simulink model "MIL4L3_SW6_V1_20220211"  (R2018b)
settings: Solver=FixedStepAuto  StartTime=0.0  StopTime=inf  FixedStep=0.001  RelTol=1e-3
PreLoadFcn:
  | A0_MILtest;
undefined symbols (not defined in the file or in its folder): Clb_ICADirect_LaneDisp_StateFive, Clb_ICADirect_LaneDisp_StateFour, Clb_ICADirect_LaneDisp_StateOne, Clb_ICADirect_LaneDisp_StateThree, Clb_ICADirect_LaneDisp_StateTwo, Clb_ICADirect_LaneDisp_StateZero, Clb_ICADirect_LaneDispSW, Clb_ICADirect_TrnLghtsCom_Switch, Clb_ICADirect_TrnLghtsCom_Value, Clb_ICADirect_TrnLghtsCrtl_Inhb, IMAP_Clb_ACU_Driver_Belt, IMAP_Clb_ACU_Driver_Belt_Over, IMAP_Clb_ACU_Passenger_Belt, IMAP_Clb_ACU_Passenger_Belt_Over, IMAP_Clb_ACU_RearLeft_Belt, IMAP_Clb_ACU_RearLeft_Belt_Over, IMAP_Clb_ACU_RearMiddle_Belt, IMAP_Clb_ACU_RearMiddle_Belt_Over, IMAP_Clb_ACU_RearRight_Belt, IMAP_Clb_ACU_RearRight_Belt_Over, IMAP_Clb_AEB_Switch, IMAP_Clb_AEB_Switch_Over, IMAP_Clb_ALC_TLC_Mode, IMAP_Clb_ALC_TLC_Mode_Over, IMAP_Clb_BCM_Battery_Voltage, IMAP_Clb_BCM_Battery_Voltage_Over, IMAP_Clb_BCM_BrakeLamp_State, IMAP_Clb_BCM_BrakeLamp_State_Over, IMAP_Clb_BCM_CHMSL_Status, IMAP_Clb_BCM_CHMSL_Status_Over, IMAP_Clb_BCM_Door_Lock_State, IMAP_Clb_BCM_Door_Lock_State_Over, IMAP_Clb_BCM_FrontWiper_State, IMAP_Clb_BCM_FrontWiper_State_Over, IMAP_Clb_BCM_FrontWiper_Switch, IMAP_Clb_BCM_FrontWiper_Switch_Over, IMAP_Clb_BCM_HazardLamp, IMAP_Clb_BCM_HazardLamp_Over, IMAP_Clb_BCM_HazardLamp_Switch, IMAP_Clb_BCM_HazardLamp_Switch_Over, IMAP_Clb_BCM_HighBeam_State, IMAP_Clb_BCM_HighBeam_State_Over, IMAP_Clb_BCM_Ignition_State, IMAP_Clb_BCM_Ignition_State_Over, IMAP_Clb_BCM_IHBC_Enabled, IMAP_Clb_BCM_IHBC_Enabled_Over, IMAP_Clb_BCM_Left_Light, IMAP_Clb_BCM_Left_Light_Over, IMAP_Clb_BCM_LeftTurn_Switch, IMAP_Clb_BCM_LeftTurn_Switch_Over, IMAP_Clb_BCM_LF_Door_State, IMAP_Clb_BCM_LF_Door_State_Over, IMAP_Clb_BCM_LowBeam_State, IMAP_Clb_BCM_LowBeam_State_Over, IMAP_Clb_BCM_LR_Door_State, IMAP_Clb_BCM_LR_Door_State_Over, IMAP_Clb_BCM_RF_Door_State, IMAP_Clb_BCM_RF_Door_State_Over, IMAP_Clb_BCM_Right_Light, IMAP_Clb_BCM_Right_Light_Over ... (+547)
libraries: CarMaker4SL x2153, simulink x292, dspstat3 x3, canmsglib x2, simulink_extras x1
(part 3 of 52)

== system MIL4L3_SW6_V1_20220211/CarMaker/VehicleControl/Radar_Define ==
  Define CM Dict : CarMaker4SL/Define CM Dict  xname=User.IO.Out.T00.dtct  xmono=off  xtype=Double4  xdvaplace=None  xnstates=0  xfirststate=0  xinitial=0
  Define CM Dict1 : CarMaker4SL/Define CM Dict  xname=User.IO.Out.T01.dtct  xmono=off  xtype=Double4  xdvaplace=None  xnstates=0  xfirststate=0  xinitial=0
  Define CM Dict10 : CarMaker4SL/Define CM Dict  xname=User.IO.Out.T02.LatDistance  xmono=off  xtype=Double4  xdvaplace=None  xnstates=0  xfirststate=0  xinitial=0
  Define CM Dict11 : CarMaker4SL/Define CM Dict  xname=User.IO.Out.T03.LatDistance  xmono=off  xtype=Double4  xdvaplace=None  xnstates=0  xfirststate=0  xinitial=0
  Define CM Dict12 : CarMaker4SL/Define CM Dict  xname=User.IO.Out.T00.RelativeLongVelo  xmono=off  xtype=Double4  xdvaplace=None  xnstates=0  xfirststate=0  xinitial=0
  Define CM Dict13 : CarMaker4SL/Define CM Dict  xname=User.IO.Out.T01.RelativeLongVelo  xmono=off  xtype=Double4  xdvaplace=None  xnstates=0  xfirststate=0  xinitial=0
  Define CM Dict14 : CarMaker4SL/Define CM Dict  xname=User.IO.Out.T02.RelativeLongVelo  xmono=off  xtype=Double4  xdvaplace=None  xnstates=0  xfirststate=0  xinitial=0
  Define CM Dict15 : CarMaker4SL/Define CM Dict  xname=User.IO.Out.T03.RelativeLongVelo  xmono=off  xtype=Double4  xdvaplace=None  xnstates=0  xfirststate=0  xinitial=0
  Define CM Dict16 : CarMaker4SL/Define CM Dict  xname=User.IO.Out.T00.RelativeLatVelo  xmono=off  xtype=Double4  xdvaplace=None  xnstates=0  xfirststate=0  xinitial=0
  Define CM Dict17 : CarMaker4SL/Define CM Dict  xname=User.IO.Out.T01.RelativeLatVelo  xmono=off  xtype=Double4  xdvaplace=None  xnstates=0  xfirststate=0  xinitial=0
  Define CM Dict18 : CarMaker4SL/Define CM Dict  xname=User.IO.Out.T02.RelativeLatVelo  xmono=off  xtype=Double4  xdvaplace=None  xnstates=0  xfirststate=0  xinitial=0
  Define CM Dict19 : CarMaker4SL/Define CM Dict  xname=User.IO.Out.T03.RelativeLatVelo  xmono=off  xtype=Double4  xdvaplace=None  xnstates=0  xfirststate=0  xinitial=0
  Define CM Dict2 : CarMaker4SL/Define CM Dict  xname=User.IO.Out.T02.dtct  xmono=off  xtype=Double4  xdvaplace=None  xnstates=0  xfirststate=0  xinitial=0
  Define CM Dict20 : CarMaker4SL/Define CM Dict  xname=User.IO.Out.T00.RelativeLatAcc  xmono=off  xtype=Double4  xdvaplace=None  xnstates=0  xfirststate=0  xinitial=0
  Define CM Dict21 : CarMaker4SL/Define CM Dict  xname=User.IO.Out.T01.RelativeLatAcc  xmono=off  xtype=Double4  xdvaplace=None  xnstates=0  xfirststate=0  xinitial=0
  Define CM Dict22 : CarMaker4SL/Define CM Dict  xname=User.IO.Out.T02.RelativeLatAcc  xmono=off  xtype=Double4  xdvaplace=None  xnstates=0  xfirststate=0  xinitial=0
  Define CM Dict23 : CarMaker4SL/Define CM Dict  xname=User.IO.Out.T03.RelativeLatAcc  xmono=off  xtype=Double4  xdvaplace=None  xnstates=0  xfirststate=0  xinitial=0
  Define CM Dict24 : CarMaker4SL/Define CM Dict  xname=User.IO.Out.T00.RelativeLongAcc  xmono=off  xtype=Double4  xdvaplace=None  xnstates=0  xfirststate=0  xinitial=0
  Define CM Dict25 : CarMaker4SL/Define CM Dict  xname=User.IO.Out.T01.RelativeLongAcc  xmono=off  xtype=Double4  xdvaplace=None  xnstates=0  xfirststate=0  xinitial=0
  Define CM Dict26 : CarMaker4SL/Define CM Dict  xname=User.IO.Out.T02.RelativeLongAcc  xmono=off  xtype=Double4  xdvaplace=None  xnstates=0  xfirststate=0  xinitial=0
  Define CM Dict27 : CarMaker4SL/Define CM Dict  xname=User.IO.Out.T03.RelativeLongAcc  xmono=off  xtype=Double4  xdvaplace=None  xnstates=0  xfirststate=0  xinitial=0
  Define CM Dict28 : CarMaker4SL/Define CM Dict  xname=User.IO.Out.T00.AbsoluteLongVelo  xmono=off  xtype=Double4  xdvaplace=None  xnstates=0  xfirststate=0  xinitial=0
  Define CM Dict29 : CarMaker4SL/Define CM Dict  xname=User.IO.Out.T01.AbsoluteLongVelo  xmono=off  xtype=Double4  xdvaplace=None  xnstates=0  xfirststate=0  xinitial=0
  Define CM Dict3 : CarMaker4SL/Define CM Dict  xname=User.IO.Out.T03.dtct  xmono=off  xtype=Double4  xdvaplace=None  xnstates=0  xfirststate=0  xinitial=0
  Define CM Dict30 : CarMaker4SL/Define CM Dict  xname=User.IO.Out.T02.AbsoluteLongVelo  xmono=off  xtype=Double4  xdvaplace=None  xnstates=0  xfirststate=0  xinitial=0
  Define CM Dict31 : CarMaker4SL/Define CM Dict  xname=User.IO.Out.T03.AbsoluteLongVelo  xmono=off  xtype=Double4  xdvaplace=None  xnstates=0  xfirststate=0  xinitial=0
  Define CM Dict32 : CarMaker4SL/Define CM Dict  xname=User.IO.Out.T00.AbsoluteLongAcc  xmono=off  xtype=Double4  xdvaplace=None  xnstates=0  xfirststate=0  xinitial=0
  Define CM Dict33 : CarMaker4SL/Define CM Dict  xname=User.IO.Out.T01.AbsoluteLongAcc  xmono=off  xtype=Double4  xdvaplace=None  xnstates=0  xfirststate=0  xinitial=0
  Define CM Dict34 : CarMaker4SL/Define CM Dict  xname=User.IO.Out.T02.AbsoluteLongAcc  xmono=off  xtype=Double4  xdvaplace=None  xnstates=0  xfirststate=0  xinitial=0
  Define CM Dict35 : CarMaker4SL/Define CM Dict  xname=User.IO.Out.T03.AbsoluteLongAcc  xmono=off  xtype=Double4  xdvaplace=None  xnstates=0  xfirststate=0  xinitial=0
  Define CM Dict36 : CarMaker4SL/Define CM Dict  xname=User.IO.Out.T00.AbsoluteLatVelo  xmono=off  xtype=Double4  xdvaplace=None  xnstates=0  xfirststate=0  xinitial=0
  Define CM Dict37 : CarMaker4SL/Define CM Dict  xname=User.IO.Out.T01.AbsoluteLatVelo  xmono=off  xtype=Double4  xdvaplace=None  xnstates=0  xfirststate=0  xinitial=0
  Define CM Dict38 : CarMaker4SL/Define CM Dict  xname=User.IO.Out.T02.AbsoluteLatVelo  xmono=off  xtype=Double4  xdvaplace=None  xnstates=0  xfirststate=0  xinitial=0
  Define CM Dict39 : CarMaker4SL/Define CM Dict  xname=User.IO.Out.T03.AbsoluteLatVelo  xmono=off  xtype=Double4  xdvaplace=None  xnstates=0  xfirststate=0  xinitial=0
  Define CM Dict4 : CarMaker4SL/Define CM Dict  xname=User.IO.Out.T00.LongDistance  xmono=off  xtype=Double4  xdvaplace=None  xnstates=0  xfirststate=0  xinitial=0
  Define CM Dict40 : CarMaker4SL/Define CM Dict  xname=User.IO.Out.T00.AbsoluteLatAcc  xmono=off  xtype=Double4  xdvaplace=None  xnstates=0  xfirststate=0  xinitial=0
  Define CM Dict41 : CarMaker4SL/Define CM Dict  xname=User.IO.Out.T01.AbsoluteLatAcc  xmono=off  xtype=Double4  xdvaplace=None  xnstates=0  xfirststate=0  xinitial=0
  Define CM Dict42 : CarMaker4SL/Define CM Dict  xname=User.IO.Out.T02.AbsoluteLatAcc  xmono=off  xtype=Double4  xdvaplace=None  xnstates=0  xfirststate=0  xinitial=0
  Define CM Dict43 : CarMaker4SL/Define CM Dict  xname=User.IO.Out.T03.AbsoluteLatAcc  xmono=off  xtype=Double4  xdvaplace=None  xnstates=0  xfirststate=0  xinitial=0
  Define CM Dict44 : CarMaker4SL/Define CM Dict  xname=User.IO.Out.T00.ClassType  xmono=off  xtype=Double4  xdvaplace=None  xnstates=0  xfirststate=0  xinitial=0
  Define CM Dict45 : CarMaker4SL/Define CM Dict  xname=User.IO.Out.T01.ClassType  xmono=off  xtype=Double4  xdvaplace=None  xnstates=0  xfirststate=0  xinitial=0
  Define CM Dict46 : CarMaker4SL/Define CM Dict  xname=User.IO.Out.T02.ClassType  xmono=off  xtype=Double4  xdvaplace=None  xnstates=0  xfirststate=0  xinitial=0
  Define CM Dict47 : CarMaker4SL/Define CM Dict  xname=User.IO.Out.T03.ClassType  xmono=off  xtype=Double4  xdvaplace=None  xnstates=0  xfirststate=0  xinitial=0
  Define CM Dict48 : CarMaker4SL/Define CM Dict  xname=User.IO.Out.T00.ClassProbValue  xmono=off  xtype=Double4  xdvaplace=None  xnstates=0  xfirststate=0  xinitial=0
  Define CM Dict49 : CarMaker4SL/Define CM Dict  xname=User.IO.Out.T01.ClassProbValue  xmono=off  xtype=Double4  xdvaplace=None  xnstates=0  xfirststate=0  xinitial=0
  Define CM Dict5 : CarMaker4SL/Define CM Dict  xname=User.IO.Out.T01.LongDistance  xmono=off  xtype=Double4  xdvaplace=None  xnstates=0  xfirststate=0  xinitial=0
  Define CM Dict50 : CarMaker4SL/Define CM Dict  xname=User.IO.Out.T02.ClassProbValue  xmono=off  xtype=Double4  xdvaplace=None  xnstates=0  xfirststate=0  xinitial=0
  Define CM Dict51 : CarMaker4SL/Define CM Dict  xname=User.IO.Out.T03.ClassProbValue  xmono=off  xtype=Double4  xdvaplace=None  xnstates=0  xfirststate=0  xinitial=0
  Define CM Dict52 : CarMaker4SL/Define CM Dict  xname=User.IO.Out.T00.Length  xmono=off  xtype=Double4  xdvaplace=None  xnstates=0  xfirststate=0  xinitial=0
  Define CM Dict53 : CarMaker4SL/Define CM Dict  xname=User.IO.Out.T01.Length  xmono=off  xtype=Double4  xdvaplace=None  xnstates=0  xfirststate=0  xinitial=0
  Define CM Dict54 : CarMaker4SL/Define CM Dict  xname=User.IO.Out.T02.Length  xmono=off  xtype=Double4  xdvaplace=None  xnstates=0  xfirststate=0  xinitial=0
  Define CM Dict55 : CarMaker4SL/Define CM Dict  xname=User.IO.Out.T03.Length  xmono=off  xtype=Double4  xdvaplace=None  xnstates=0  xfirststate=0  xinitial=0
  Define CM Dict56 : CarMaker4SL/Define CM Dict  xname=User.IO.Out.T00.Widh  xmono=off  xtype=Double4  xdvaplace=None  xnstates=0  xfirststate=0  xinitial=0
  Define CM Dict57 : CarMaker4SL/Define CM Dict  xname=User.IO.Out.T01.Widh  xmono=off  xtype=Double4  xdvaplace=None  xnstates=0  xfirststate=0  xinitial=0
  Define CM Dict58 : CarMaker4SL/Define CM Dict  xname=User.IO.Out.T02.Widh  xmono=off  xtype=Double4  xdvaplace=None  xnstates=0  xfirststate=0  xinitial=0
  Define CM Dict59 : CarMaker4SL/Define CM Dict  xname=User.IO.Out.T03.Widh  xmono=off  xtype=Double4  xdvaplace=None  xnstates=0  xfirststate=0  xinitial=0
  Define CM Dict6 : CarMaker4SL/Define CM Dict  xname=User.IO.Out.T02.LongDistance  xmono=off  xtype=Double4  xdvaplace=None  xnstates=0  xfirststate=0  xinitial=0
  Define CM Dict60 : CarMaker4SL/Define CM Dict  xname=User.IO.Out.T00.Height  xmono=off  xtype=Double4  xdvaplace=None  xnstates=0  xfirststate=0  xinitial=0
  Define CM Dict61 : CarMaker4SL/Define CM Dict  xname=User.IO.Out.T01.Height  xmono=off  xtype=Double4  xdvaplace=None  xnstates=0  xfirststate=0  xinitial=0
  Define CM Dict62 : CarMaker4SL/Define CM Dict  xname=User.IO.Out.T02.Height  xmono=off  xtype=Double4  xdvaplace=None  xnstates=0  xfirststate=0  xinitial=0
  Define CM Dict63 : CarMaker4SL/Define CM Dict  xname=User.IO.Out.T03.Height  xmono=off  xtype=Double4  xdvaplace=None  xnstates=0  xfirststate=0  xinitial=0
  Define CM Dict64 : CarMaker4SL/Define CM Dict  xname=User.IO.Out.T00.ObjectID  xmono=off  xtype=Double4  xdvaplace=None  xnstates=0  xfirststate=0  xinitial=0
  Define CM Dict65 : CarMaker4SL/Define CM Dict  xname=User.IO.Out.T01.ObjectID  xmono=off  xtype=Double4  xdvaplace=None  xnstates=0  xfirststate=0  xinitial=0
  Define CM Dict66 : CarMaker4SL/Define CM Dict  xname=User.IO.Out.T02.ObjectID  xmono=off  xtype=Double4  xdvaplace=None  xnstates=0  xfirststate=0  xinitial=0
  Define CM Dict67 : CarMaker4SL/Define CM Dict  xname=User.IO.Out.T03.ObjectID  xmono=off  xtype=Double4  xdvaplace=None  xnstates=0  xfirststate=0  xinitial=0
  Define CM Dict68 : CarMaker4SL/Define CM Dict  xname=User.IO.Out.T00.YawAngle  xmono=off  xtype=Double4  xdvaplace=None  xnstates=0  xfirststate=0  xinitial=0
  Define CM Dict69 : CarMaker4SL/Define CM Dict  xname=User.IO.Out.T01.YawAngle  xmono=off  xtype=Double4  xdvaplace=None  xnstates=0  xfirststate=0  xinitial=0
  Define CM Dict7 : CarMaker4SL/Define CM Dict  xname=User.IO.Out.T03.LongDistance  xmono=off  xtype=Double4  xdvaplace=None  xnstates=0  xfirststate=0  xinitial=0
  Define CM Dict70 : CarMaker4SL/Define CM Dict  xname=User.IO.Out.T02.YawAngle  xmono=off  xtype=Double4  xdvaplace=None  xnstates=0  xfirststate=0  xinitial=0
  Define CM Dict71 : CarMaker4SL/Define CM Dict  xname=User.IO.Out.T03.YawAngle  xmono=off  xtype=Double4  xdvaplace=None  xnstates=0  xfirststate=0  xinitial=0
  Define CM Dict72 : CarMaker4SL/Define CM Dict  xname=User.IO.Out.T00.MovementStatus  xmono=off  xtype=Double4  xdvaplace=None  xnstates=0  xfirststate=0  xinitial=0
  Define CM Dict73 : CarMaker4SL/Define CM Dict  xname=User.IO.Out.T01.MovementStatus  xmono=off  xtype=Double4  xdvaplace=None  xnstates=0  xfirststate=0  xinitial=0
  Define CM Dict74 : CarMaker4SL/Define CM Dict  xname=User.IO.Out.T02.MovementStatus  xmono=off  xtype=Double4  xdvaplace=None  xnstates=0  xfirststate=0  xinitial=0
  Define CM Dict75 : CarMaker4SL/Define CM Dict  xname=User.IO.Out.T03.MovementStatus  xmono=off  xtype=Double4  xdvaplace=None  xnstates=0  xfirststate=0  xinitial=0
  Define CM Dict76 : CarMaker4SL/Define CM Dict  xname=User.IO.Out.T00.MeasurementStatus  xmono=off  xtype=Double4  xdvaplace=None  xnstates=0  xfirststate=0  xinitial=0
  Define CM Dict77 : CarMaker4SL/Define CM Dict  xname=User.IO.Out.T01.MeasurementStatus  xmono=off  xtype=Double4  xdvaplace=None  xnstates=0  xfirststate=0  xinitial=0
  Define CM Dict78 : CarMaker4SL/Define CM Dict  xname=User.IO.Out.T02.MeasurementStatus  xmono=off  xtype=Double4  xdvaplace=None  xnstates=0  xfirststate=0  xinitial=0
  Define CM Dict79 : CarMaker4SL/Define CM Dict  xname=User.IO.Out.T03.MeasurementStatus  xmono=off  xtype=Double4  xdvaplace=None  xnstates=0  xfirststate=0  xinitial=0
  Define CM Dict8 : CarMaker4SL/Define CM Dict  xname=User.IO.Out.T00.LatDistance  xmono=off  xtype=Double4  xdvaplace=None  xnstates=0  xfirststate=0  xinitial=0
  Define CM Dict80 : CarMaker4SL/Define CM Dict  xname=User.IO.Out.T00.TimeStamp  xmono=off  xtype=Double4  xdvaplace=None  xnstates=0  xfirststate=0  xinitial=0
  Define CM Dict81 : CarMaker4SL/Define CM Dict  xname=User.IO.Out.T01.TimeStamp  xmono=off  xtype=Double4  xdvaplace=None  xnstates=0  xfirststate=0  xinitial=0
  Define CM Dict82 : CarMaker4SL/Define CM Dict  xname=User.IO.Out.T02.TimeStamp  xmono=off  xtype=Double4  xdvaplace=None  xnstates=0  xfirststate=0  xinitial=0
  Define CM Dict83 : CarMaker4SL/Define CM Dict  xname=User.IO.Out.T03.TimeStamp  xmono=off  xtype=Double4  xdvaplace=None  xnstates=0  xfirststate=0  xinitial=0
  Define CM Dict84 : CarMaker4SL/Define CM Dict  xname=User.IO.Out.T00.ExistenceProb  xmono=off  xtype=Double4  xdvaplace=None  xnstates=0  xfirststate=0  xinitial=0
  Define CM Dict85 : CarMaker4SL/Define CM Dict  xname=User.IO.Out.T01.ExistenceProb  xmono=off  xtype=Double4  xdvaplace=None  xnstates=0  xfirststate=0  xinitial=0
  Define CM Dict86 : CarMaker4SL/Define CM Dict  xname=User.IO.Out.T02.ExistenceProb  xmono=off  xtype=Double4  xdvaplace=None  xnstates=0  xfirststate=0  xinitial=0
  Define CM Dict87 : CarMaker4SL/Define CM Dict  xname=User.IO.Out.T03.ExistenceProb  xmono=off  xtype=Double4  xdvaplace=None  xnstates=0  xfirststate=0  xinitial=0
  Define CM Dict9 : CarMaker4SL/Define CM Dict  xname=User.IO.Out.T01.LatDistance  xmono=off  xtype=Double4  xdvaplace=None  xnstates=0  xfirststate=0  xinitial=0
